simulink model "MAP_TEST"  (R2022a)
settings: Solver=FixedStepDiscrete  StartTime=0.0  StopTime=200  FixedStep=0.04  RelTol=1e-3
PreLoadFcn:
  | addpath('C:\Users\ASCL\Documents\GitHub\DTNS\MAP');
  | addpath('C:\Users\ASCL\Documents\GitHub\DTNS\MAP_DB\');
  | addpath('MAP');
InitFcn:
  | addpath('C:\Users\ASCL\Documents\GitHub\DTNS\MAP');
  | addpath('C:\Users\ASCL\Documents\GitHub\DTNS\MAP_DB\');
  | addpath('MAP');
settings Model: Creator=ASCL  LastModifiedBy=ASCL
settings DataIOCC: SaveOutput=off  SignalLogging=off  DSMLogging=off  SaveTime=off  ReturnWorkspaceOutputs=off
settings OptimizationCC: BlockReduction=off  DefaultParameterBehavior=Inlined  UseDivisionForNetSlopeComputation=on  GainParamInheritBuiltInType=on  UseFloatMulNetSlope=on  ExpressionFolding=off  PassReuseOutputArgsAs=Individual arguments  ZeroExternalMemoryAtStartup=off  ZeroInternalMemoryAtStartup=off  EfficientFloat2IntCast=on  LifeSpan=inf  OptimizeBlockOrder=speed  DifferentSizesBufferReuse=on  EfficientTunableParamExpr=on
settings DebuggingCC: SignalInfNanChecking=warning  ReadBeforeWriteMsg=EnableAllAsError  WriteAfterWriteMsg=EnableAllAsError  WriteAfterReadMsg=EnableAllAsError  IntegerOverflowMsg=error  ParameterTunabilityLossMsg=error  UniqueDataStoreMsg=error  AssertControl=DisableAll  NonBusSignalsTreatedAsBus=error  SFInvalidInputDataAccessInChartInitDiag=error  SFTransitionOutsideNaturalParentDiag=error  SFUnreachableExecutionPathDiag=error  SFUndirectedBroadcastEventsDiag=error  IntegerSaturationMsg=error
settings HardwareCC: ProdBitPerPointer=32  ProdBitPerSizeT=32  ProdBitPerPtrDiffT=32  ProdLargestAtomicInteger=Long  ProdLargestAtomicFloat=Double  ProdEndianess=BigEndian  ProdWordSize=32  ProdLongLongMode=on  ProdHWDeviceType=Freescale->MPC83xx
settings ModelReferenceCC: ModelReferenceNumInstancesAllowed=Single
settings SFSimCC: SimCustomHeaderCode="#include \"MAP.h\""  SimUserSources=MAP.c  SimUserLibraries=WS2_32.LIB  CompileTimeRecursionLimit=0  EnableRuntimeRecursion=off  MATLABDynamicMemAlloc=off
settings RTWCC: SystemTargetFile=ert.tlc  TemplateMakefile=ert_default_tmf  GenerateReport=on  RTWUseSimCustomCode=on  CustomHeaderCode="#include \"MAP.h\""  CustomSource=MAP.c  CustomLibrary=WS2_32.LIB  BuildConfiguration=Faster Runs  IncludeHyperlinkInReport=on  LaunchReport=on  GenerateTraceInfo=on  GenerateTraceReport=on  GenerateTraceReportSl=on  GenerateTraceReportSf=on  GenerateTraceReportEml=on
settings CodeAppCC: ForceParamTrailComments=on  IgnoreCustomStorageClasses=off  OperatorAnnotations=on  SimulinkDataObjDesc=on  SFDataObjDesc=on  MATLABFcnDesc=on  InsertBlockDesc=on  StateflowObjectComments=on  MATLABSourceComments=on  EnableCustomComments=on  InlinedPrmAccess=Macros  ReqsInCode=on
settings ERTTargetCC: TargetLangStandard=C99 (ISO)  UtilityFuncGeneration=Shared location  GenerateSampleERTMain=on  IncludeMdlTerminateFcn=off  CombineSignalStateStructs=on  SuppressErrorStatus=on  SupportAbsoluteTime=off  SupportNonFinite=off  SupportComplex=off  ParenthesesLevel=Standards  CastingMode=Standards  GenerateSharedConstants=off  InlinedParameterPlacement=NonHierarchical  ERTCustomFileTemplate=example_file_process.tlc  RateTransitionBlockCode=Function  PreserveIfCondition=on  ConvertIfToSwitch=off  EnableSignedLeftShifts=off  EnableSignedRightShifts=off

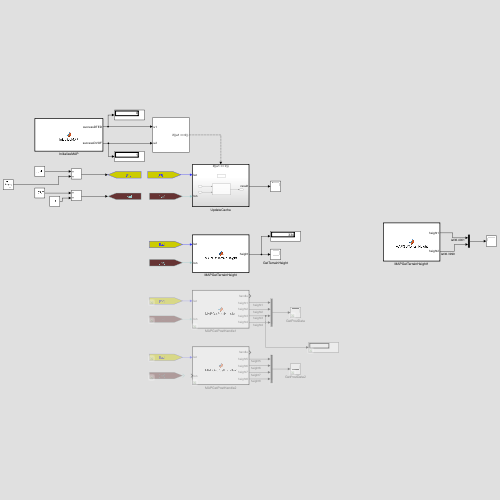
[thumbnail: Simulink's stored preview of the top-level diagram]
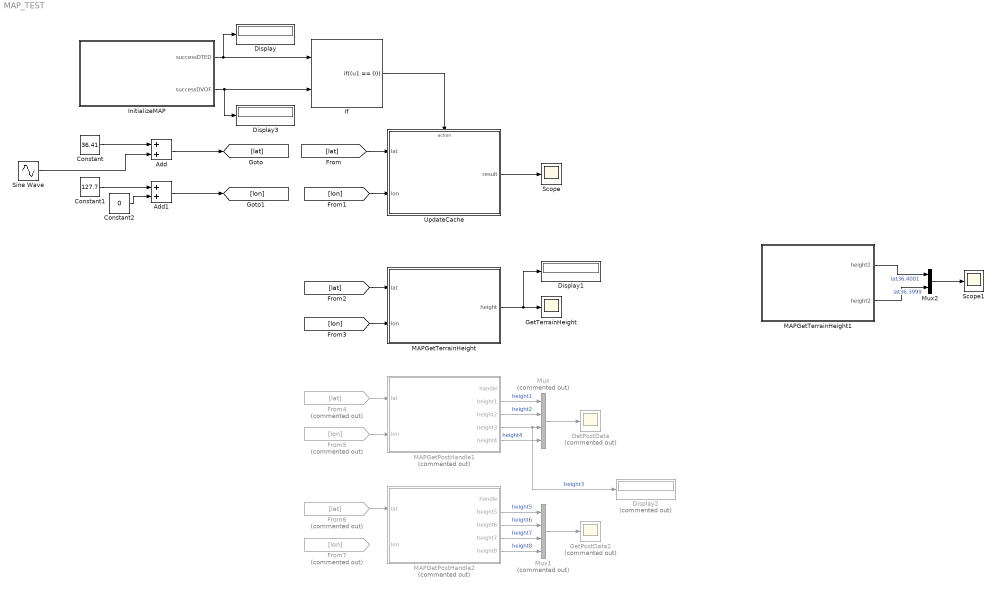
== system MAP_TEST ==
  Add : Sum
  Add1 : Sum
  Constant : Constant  Value=36.41
  Constant1 : Constant  Value=127.7
  Constant2 : Constant  Value=0
  Display : Display
  Display1 : Display
  Display2 : Display  Commented=on
  Display3 : Display
  From4 : From  Commented=on  GotoTag=lat
  From5 : From  Commented=on  GotoTag=lon
  From6 : From  Commented=on  GotoTag=lat
  From7 : From  Commented=on  GotoTag=lon
  GetPostData : Scope  Commented=on
  GetPostData2 : Scope  Commented=on
  GetTerrainHeight : Scope
  If : If  NumInputs=2  IfExpression=(u1 == 0)  ShowElse=off
  InitializeMAP : MATLAB Function  TreatAsAtomicUnit=on
  MAPGetPostHandle1 : MATLAB Function  Commented=on  TreatAsAtomicUnit=on
  MAPGetPostHandle2 : MATLAB Function  Commented=on  TreatAsAtomicUnit=on
  MAPGetTerrainHeight : MATLAB Function  TreatAsAtomicUnit=on
  MAPGetTerrainHeight1 : MATLAB Function  TreatAsAtomicUnit=on
  Mux : Mux  Commented=on
  Mux1 : Mux  Commented=on
  Mux2 : Mux  Inputs=2
  Scope : Scope
  Scope1 : Scope
  Sine Wave : Sin  Amplitude=0  Frequency=0.5  SampleTime=0.04
  UpdateCache : Subsystem  TreatAsAtomicUnit=on
  wires:
  Add1/1 -> [lon]
  Add/1 -> [lat]
  Constant/1 -> Add/1
  Constant1/1 -> Add1/1
  InitializeMAP/1(successDTED) -> Display/1, If/1
  InitializeMAP/2(successDVOF) -> Display3/1, If/2
  If/1 -> UpdateCache/Action
  UpdateCache/1(result) -> Scope/1
  [lon] -> UpdateCache/2(lon)
  [lat] -> UpdateCache/1(lat)
  [lat] -> MAPGetTerrainHeight/1(lat)
  [lon] -> MAPGetTerrainHeight/2(lon)
  MAPGetTerrainHeight/1(height) -> Display1/1, GetTerrainHeight/1
  Constant2/1 -> Add1/2
  From4/1 -> MAPGetPostHandle1/1(lat)
  From5/1 -> MAPGetPostHandle1/2(lon)
  MAPGetPostHandle1/2(height1) -> Mux/1  "height1"
  MAPGetPostHandle1/3(height2) -> Mux/2  "height2"
  MAPGetPostHandle1/4(height3) -> Display2/1, Mux/3  "height3"
  MAPGetPostHandle1/5(height4) -> Mux/4  "height4"
  Mux/1 -> GetPostData/1
  From6/1 -> MAPGetPostHandle2/1(lat)
  MAPGetPostHandle2/2(height5) -> Mux1/1  "height5"
  MAPGetPostHandle2/3(height6) -> Mux1/2  "height6"
  MAPGetPostHandle2/4(height7) -> Mux1/3  "height7"
  MAPGetPostHandle2/5(height8) -> Mux1/4  "height8"
  Mux1/1 -> GetPostData2/1
  Sine Wave/1 -> Add/2
  Mux2/1 -> Scope1/1
  MAPGetTerrainHeight1/1(height1) -> Mux2/1  "lat36.4001"
  MAPGetTerrainHeight1/2(height2) -> Mux2/2  "lat36.3999"

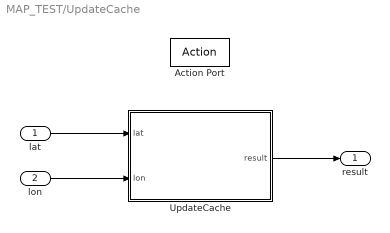
== system MAP_TEST/UpdateCache ==
  lat : Inport
  lon : Inport  Port=2
  Action Port : ActionPort  ActionPortLabel=if((u1 == 0))
  UpdateCache : MATLAB Function  TreatAsAtomicUnit=on
  result : Outport
  wires:
  UpdateCache/1(result) -> result/1
  lat/1 -> UpdateCache/1(lat)
  lon/1 -> UpdateCache/2(lon)

== matlab function MAP_TEST/InitializeMAP ==
  data: successDTED output; successDVOF output
function [successDTED, successDVOF] = InitializeMAP()
%InitializeMAP

% Persistent variable
persistent firstRun
if isempty(firstRun)
    firstRun = true;
end

% Initialize output
flagDTED = int32(1);
flagDVOF = int32(1);
successDTED = int32(1);
successDVOF = int32(1);

if firstRun
    % Path of DTED data
    pathDTED = 'C:\Users\ASCL\Documents\GitHub\DTNS\MAP\MAP_DB';

    % Length of DETD data path
    strLenDTED = int32(strlength(pathDTED));
    
    % Call [ InitialMap ] : 맵 폴더 위치 설정
    flagDTED = coder.ceval('InitialMap', pathDTED, strLenDTED );
    
    successDTED = flagDTED;

    if (successDTED)
        firstRun = false;
    end
else
    successDTED = int32(0);
    successDVOF = int32(0);
end

== matlab function MAP_TEST/UpdateCache/UpdateCache ==
  data: result output; lat input; lon input
function result = UpdateCache(lat, lon)
%UpdateCache

% Persistent variables
persistent latPrev lonPrev
if isempty(latPrev)
    latPrev = 0.0;
end
if isempty(lonPrev)
    lonPrev = 0.0;
end

% Initialize output
result = int32(1);

% if ( abs(lat - latPrev) > 0.05 ) || ( abs(lon - lonPrev) > 0.05)
    result = coder.ceval('UpdateCache', lat, lon);
    latPrev = lat;
    lonPrev = lon;
% else
    
end

== matlab function MAP_TEST/MAPGetTerrainHeight ==
  data: lat input; height output; lon input
function height = MAPGetTerrainHeight(lat, lon)
%MAPGetTerrainHeight

% Initialize
height = 0.0;

height = coder.ceval('MAPGetTerrainHeight', lat, lon);

== matlab function MAP_TEST/MAPGetPostHandle1 ==
  data: lat input; handle output; lon input; height1 output; height2 output; height3 output; height4 output
function [handle, height1, height2, height3, height4] = MAPGetPostHandle1(lat, lon)
%MAPGetPostHandle1

% Initialize
handle = int32(0);
height1 = int16(0);
height2 = int16(0);
height3 = int16(0);
height4 = int16(0);

handle = coder.ceval('MAPGetPostHandle', 0, lat, lon);
height1 = coder.ceval('MAPGetPostData', handle, 0, 0);
height2 = coder.ceval('MAPGetPostData', handle, 1, 1);
height3 = coder.ceval('MAPGetPostData', handle, 0, 10);
height4 = coder.ceval('MAPGetPostData', handle, 1, -2);

== matlab function MAP_TEST/MAPGetPostHandle2 ==
  data: lat input; handle output; lon input; height5 output; height6 output; height7 output; height8 output
function [handle, height5, height6, height7, height8] = MAPGetPostHandle2(lat, lon)
%MAPGetPostHandle2

% Initialize
handle = int32(0);
height5 = int16(0);
height6 = int16(0);
height7 = int16(0);
height8 = int16(0);

handle = coder.ceval('MAPGetPostHandle', 1, lat, lon);
height5 = coder.ceval('MAPGetPostData', handle, 0, 0);
height6 = coder.ceval('MAPGetPostData', handle, 1, 1);
height7 = coder.ceval('MAPGetPostData', handle, 0, 10);
height8 = coder.ceval('MAPGetPostData', handle, 1, -2);

== matlab function MAP_TEST/MAPGetTerrainHeight1 ==
  data: height1 output; height2 output
function [height1, height2] = MAPGetTerrainHeight
%MAPGetTerrainHeight

% Initialize
height1 = 0.0;
height2 = 0.0;

height1 = coder.ceval('MAPGetTerrainHeight', 36.4001, 127.70);
height2 = coder.ceval('MAPGetTerrainHeight', 36.3999, 127.70);
